simulink library "LimiterBtc"  (R2022b)
settings: Solver=VariableStepAuto  StartTime=0.0  StopTime=10.0  RelTol=1e-3
undefined symbols (not defined in the file or in its folder): Column
libraries: TuneVar x15, TOP x8, AudioStats x1, FeaturePath x1, HandyTextFile x1
settings Model: Creator=db1045444  LastModifiedBy=kl13806
settings SolverCC: AlgebraicLoopSolver=TrustRegion
settings DebuggingCC: UnconnectedInputMsg=warning  UnconnectedOutputMsg=warning  UnconnectedLineMsg=warning  SFMachineParentedDataDiag=warning
settings ModelReferenceCC: EnableRefExpFcnMdlSchedulingChecks=on
settings RTWCC: DLArmComputeVersion=19.05

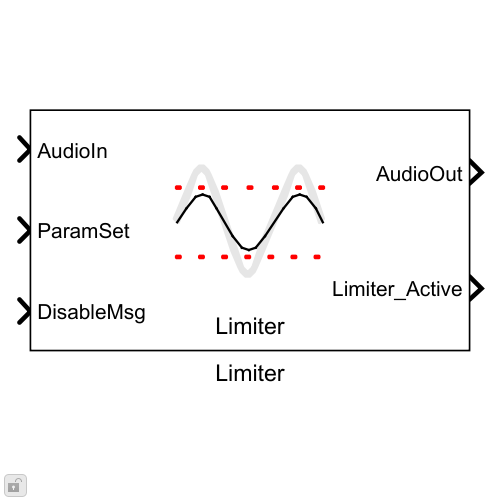
[thumbnail: Simulink's stored preview of the top-level diagram]
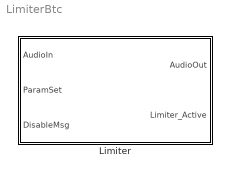
== system LimiterBtc ==
  Limiter : Subsystem  mask(Blocklib Limiter){Config=[], FeatureName=Limiter}
      mask prompts: Config "LimiterConfig"; FeatureName "Feature path name:"
      mask init:
      | blkh=gcbh;
      | Config=BTConfig.Assert(blkh,Config);
      | 
      | Config.Validate();
      | BTConfig.InitSetFeatureIfPresent(blkh,'FeatureName');
      mask Callback Config: BTConfig.CallbackHideIfPresent(gcbh,{'FeatureName'});
      mask TypeOptions FeatureName: FeaturePath/FeatureName
      mask Display:
      | [path,w,h] = IconLimiterMask();
      | 
      | % work in pixels since the icon does not scale
      | pos = get(gcbh,'position');
      | bw = pos(3) - pos(1);
      | bh = pos(4) - pos(2);
      | 
      | % Draw centered icon
      | xAdj = bw/2 - w/2;
      | yAdj = bh/2 - h/2 + 4;
      | for i=1:length(path)
      |     if (path(i).rgb(1) >= 0)
      |         patch(path(i).x+xAdj, path(i).y+yAdj, path(i).rgb);
      |     end
      |     if (path(i).stroke(1) >= 0)
      |         plot(path(i).x+xAdj, path(i).y+yAdj);
      |     end
      | end
      | 
      | % Display some text
      | text(bw/2, 4,FeatureName, ...
      |     'horizontalAlignment','center', ...
      |     'VerticalAlignment','bottom');

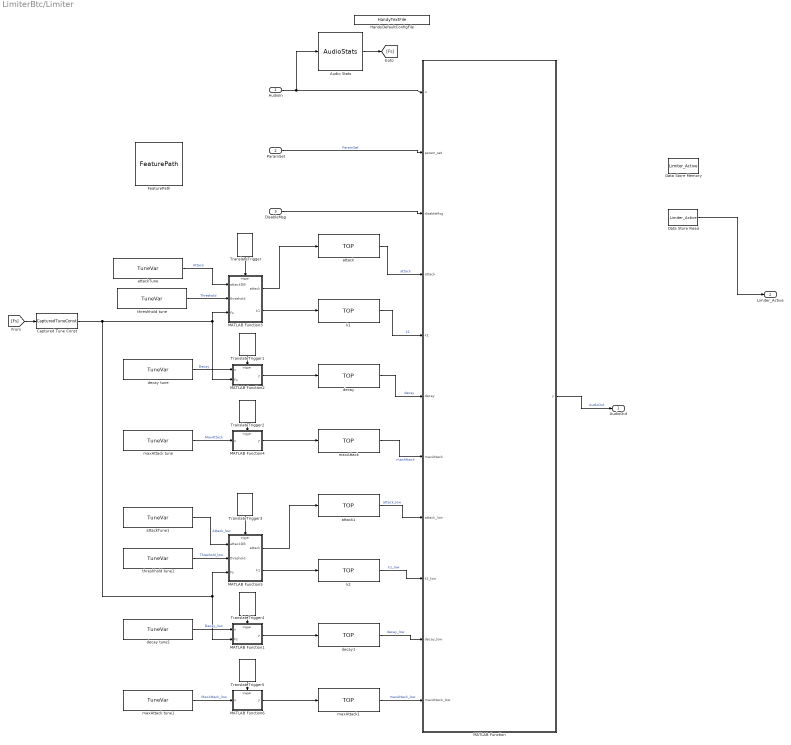
== system LimiterBtc/Limiter ==
  AudioIn : Inport
  ParamSet : Inport  Port=2
  DisableMsg : Inport  Port=3
  Audio Stats : AudioStats/AudioStats  DoSampleRate=on  TypeSampleRate=double  DoCallRate=off  TypeCallRate=Inherit: auto  DoFrameSize=off  TypeFrameSize=Inherit: auto  DoChannelCount=off  TypeChannelCount=single  DoTaskRateFactor=off  TypeTaskRateFactor=Inherit: auto  MacroNameRoot=AUDIO  MacroNameRootEval='AUDIO'  IsMacroNameEval=off  MacroSampleRate=off  MacroCallRate=off  MacroFrameSize=off  MacroChannelCount=off  MacroTaskRateFactor=off  MacroTaskId=off  ValidateSampleRate=off  ValueSampleRate=[]  ValidateCallRate=off  ValueCallRate=[]  ValidateFrameSize=off  ValueFrameSize=[]  ValidateChannelCount=off  ValueChannelCount=[]  ValidateTaskRateFactor=off  ValueTaskRateFactor=[]
      settings: SourceProductName=Bose Talaria
  Captured Tune Const : TuneVar/CapturedTuneConst  TriggerInit=[-235 487 -135 523]  Role=Automatic
      settings: SourceProductName=Bose Talaria
  Data Store Memory : DataStoreMemory  DataStoreName=Limiter_Active  ShowAdditionalParam=off  OutDataTypeStr=uint32
  Data Store Read : DataStoreRead  DataStoreName=Limiter_Active  IndexOptions=Index vector (dialog)  Indices=1  OutputSizes=1
  FeaturePath : FeaturePath/FeaturePath  FeatureName=Limiter  IsGroup=off  GroupNumber=-1  IsModule=off  TriggerInit=[10 64 125 171]
      settings: SourceProductName=Bose Talaria
  HandyDefaultConfigFile : HandyTextFile/HandyTextFile  TemplateSource=Config  FileSuffix=Init  OpenDialogOnLoad=off  UseThisBlockName=off  AddGrandParentNamePrefix=off  TheDefaultText=|  ShowInLibBrowser=on
      | % $(FILENAME) Setup model parameters for each "Init" callback (e.g. update diagram)
      | sample_rate_in_hertz = 44100;
      | frame_size = 32;
      | sysin_channel_count = 2;
      settings: SourceProductName=Bose Talaria
  MATLAB Function : MATLAB Function  TreatAsAtomicUnit=on
  MATLAB Function1 : MATLAB Function  TreatAsAtomicUnit=on
  MATLAB Function2 : MATLAB Function  TreatAsAtomicUnit=on
  MATLAB Function3 : MATLAB Function  TreatAsAtomicUnit=on
  MATLAB Function4 : MATLAB Function  TreatAsAtomicUnit=on
  MATLAB Function5 : MATLAB Function  TreatAsAtomicUnit=on
  MATLAB Function6 : MATLAB Function  TreatAsAtomicUnit=on
  TranslateTrigger : TuneVar/TranslateTrigger  TriggerInit=[261 290 299 345]
      settings: SourceProductName=Bose Talaria
  TranslateTrigger1 : TuneVar/TranslateTrigger  TriggerInit=[266 535 304 590]
      settings: SourceProductName=Bose Talaria
  TranslateTrigger2 : TuneVar/TranslateTrigger  TriggerInit=[266 700 304 755]
      settings: SourceProductName=Bose Talaria
  TranslateTrigger3 : TuneVar/TranslateTrigger  TriggerInit=[261 930 299 985]
      settings: SourceProductName=Bose Talaria
  TranslateTrigger4 : TuneVar/TranslateTrigger  TriggerInit=[266 1175 304 1230]
      settings: SourceProductName=Bose Talaria
  TranslateTrigger5 : TuneVar/TranslateTrigger  TriggerInit=[266 1340 304 1395]
      settings: SourceProductName=Bose Talaria
  attack : TOP/TOP  TriggerInit=[460 292 610 348]  TopName=attack  DataType=single  BankNumber=0  PreOverlay=false  PostOverlay=false  Role=Automatic
      settings: SourceProductName=Bose Talaria
  attack1 : TOP/TOP  TriggerInit=[460 932 610 988]  TopName=attack_low  DataType=single  BankNumber=0  PreOverlay=false  PostOverlay=false  Role=Automatic
      settings: SourceProductName=Bose Talaria
  attackTune : TuneVar/TuneVar  TuneName=Attack  SpecifyMaxSize=off  VariableDim=2 (Column)  MaxSize=[1 16]  TunabilityNumber=1  MinValue=[]  MaxValue=[]  TriggerInit=[-45 350 125 400]  MaskValue=Config.DefaultAttackDb
      settings: SourceProductName=Bose Talaria
  attackTune1 : TuneVar/TuneVar  TuneName=Attack_low  SpecifyMaxSize=off  VariableDim=2 (Column)  MaxSize=[1 1]  TunabilityNumber=1  MinValue=[]  MaxValue=[]  TriggerInit=[-20 965 150 1015]  MaskValue=Config.DefaultAttackLowDb
      settings: SourceProductName=Bose Talaria
  decay : TOP/TOP  TriggerInit=[460 612 610 668]  TopName=decay  DataType=single  BankNumber=0  PreOverlay=false  PostOverlay=false  Role=Automatic
      settings: SourceProductName=Bose Talaria
  decay tune : TuneVar/TuneVar  TuneName=Decay  SpecifyMaxSize=off  VariableDim=2 (Column)  MaxSize=[1 1]  TunabilityNumber=1  MinValue=[]  MaxValue=[]  TriggerInit=[-20 600 150 650]  MaskValue=Config.DefaultDecayDB
      settings: SourceProductName=Bose Talaria
  decay tune1 : TuneVar/TuneVar  TuneName=Decay_low  SpecifyMaxSize=off  VariableDim=2 (Column)  MaxSize=[1 1]  TunabilityNumber=1  MinValue=[]  MaxValue=[]  TriggerInit=[-20 1240 150 1290]  MaskValue=Config.DefaultDecayLowDb
      settings: SourceProductName=Bose Talaria
  decay1 : TOP/TOP  TriggerInit=[460 1252 610 1308]  TopName=decay_low  DataType=single  BankNumber=0  PreOverlay=false  PostOverlay=false  Role=Automatic
      settings: SourceProductName=Bose Talaria
  k1 : TOP/TOP  TriggerInit=[460 452 610 508]  TopName=k1  DataType=single  BankNumber=0  PreOverlay=false  PostOverlay=false  Role=Automatic
      settings: SourceProductName=Bose Talaria
  k2 : TOP/TOP  TriggerInit=[460 1092 610 1148]  TopName=k1_low  DataType=single  BankNumber=0  PreOverlay=false  PostOverlay=false  Role=Automatic
      settings: SourceProductName=Bose Talaria
  maxAttack : TOP/TOP  TriggerInit=[460 772 610 828]  TopName=maxAttack  DataType=single  BankNumber=0  PreOverlay=false  PostOverlay=false  Role=Automatic
      settings: SourceProductName=Bose Talaria
  maxAttack tune : TuneVar/TuneVar  TuneName=MaxAttack  SpecifyMaxSize=off  VariableDim=2 (Column)  MaxSize=[1 1]  TunabilityNumber=1  MinValue=[]  MaxValue=[]  TriggerInit=[-20 775 150 825]  MaskValue=Config.DefaultMaxAttackDb
      settings: SourceProductName=Bose Talaria
  maxAttack tune1 : TuneVar/TuneVar  TuneName=MaxAttack_low  SpecifyMaxSize=off  VariableDim=2 (Column)  MaxSize=[1 1]  TunabilityNumber=1  MinValue=[]  MaxValue=[]  TriggerInit=[-20 1415 150 1465]  MaskValue=Config.DefaultMaxAttackLowDb
      settings: SourceProductName=Bose Talaria
  maxAttack1 : TOP/TOP  TriggerInit=[460 1412 610 1468]  TopName=maxAttack_low  DataType=single  BankNumber=0  PreOverlay=false  PostOverlay=false  Role=Automatic
      settings: SourceProductName=Bose Talaria
  threshhold tune : TuneVar/TuneVar  TuneName=Threshold  SpecifyMaxSize=off  VariableDim=2 (Column)  MaxSize=[1 16]  TunabilityNumber=1  MinValue=[]  MaxValue=[]  TriggerInit=[-35 425 135 475]  MaskValue=Config.DefaultThreshold
      settings: SourceProductName=Bose Talaria
  threshhold tune1 : TuneVar/TuneVar  TuneName=Threshold_low  SpecifyMaxSize=off  VariableDim=2 (Column)  MaxSize=[1 1]  TunabilityNumber=1  MinValue=[]  MaxValue=[]  TriggerInit=[-20 1065 150 1115]  MaskValue=Config.DefaultThresholdLow
      settings: SourceProductName=Bose Talaria
  AudioOut : Outport  VectorParamsAs1DForOutWhenUnconnected=off
  Limiter_Active : Outport  Port=2
  wires:
  Data Store Read/1 -> Limiter_Active/1
  DisableMsg/1 -> MATLAB Function/3(disableMsg)
  AudioIn/1 -> Audio Stats/1, MATLAB Function/1(u)
  MATLAB Function/1(y) -> AudioOut/1  "AudioOut"
  attackTune/1 -> MATLAB Function3/1(attackDB)  "Attack"
  decay tune/1 -> MATLAB Function2/1(u)  "Decay"
  TranslateTrigger1/1 -> MATLAB Function2/Trigger
  attack/1 -> MATLAB Function/4(attack)  "attack"
  MATLAB Function2/1(y) -> decay/1
  decay/1 -> MATLAB Function/6(decay)  "decay"
  Audio Stats/1 -> [Fs]
  [Fs] -> Captured Tune Const/1
  threshhold tune/1 -> MATLAB Function3/2(threshold)  "Threshold"
  TranslateTrigger/1 -> MATLAB Function3/Trigger
  MATLAB Function3/2(k1) -> k1/1
  k1/1 -> MATLAB Function/5(k1)  "k1"
  maxAttack tune/1 -> MATLAB Function4/1(u)  "MaxAttack"
  TranslateTrigger2/1 -> MATLAB Function4/Trigger
  MATLAB Function4/1(y) -> maxAttack/1
  maxAttack/1 -> MATLAB Function/7(maxAttack)  "maxAttack"
  MATLAB Function3/1(attack) -> attack/1
  MATLAB Function5/1(attack) -> attack1/1
  maxAttack1/1 -> MATLAB Function/11(maxAttack_low)  "maxAttack_low"
  MATLAB Function6/1(y) -> maxAttack1/1
  TranslateTrigger5/1 -> MATLAB Function6/Trigger
  Captured Tune Const/1 -> MATLAB Function3/3(Fs), MATLAB Function2/2(Fs), MATLAB Function5/3(Fs), MATLAB Function1/2(Fs)
  MATLAB Function1/1(y) -> decay1/1
  decay1/1 -> MATLAB Function/10(decay_low)  "decay_low"
  decay tune1/1 -> MATLAB Function1/1(u)  "Decay_low"
  k2/1 -> MATLAB Function/9(k1_low)  "k1_low"
  attackTune1/1 -> MATLAB Function5/1(attackDB)  "Attack_low"
  threshhold tune1/1 -> MATLAB Function5/2(threshold)  "Threshold_low"
  MATLAB Function5/2(k1) -> k2/1
  TranslateTrigger3/1 -> MATLAB Function5/Trigger
  maxAttack tune1/1 -> MATLAB Function6/1(u)  "MaxAttack_low"
  TranslateTrigger4/1 -> MATLAB Function1/Trigger
  attack1/1 -> MATLAB Function/8(attack_low)  "attack_low"
  ParamSet/1 -> MATLAB Function/2(param_set)  "ParamSet"

== matlab function LimiterBtc/Limiter/MATLAB Function1 ==
  data: u input; y output; Fs input
  events: trigger input FUNCTION_CALL_EVENT
function y = fcn(u, Fs)

% Convert from dB to linear
y = single(undb20(abs(u.Value) / Fs));

== matlab function LimiterBtc/Limiter/MATLAB Function ==
  data: u input; param_set input; disableMsg input; y output; attack input; k1 input; decay input; maxAttack input; attack_low input; k1_low input; decay_low input; maxAttack_low input; Limiter_Active data_store_memory
function y = limiter(u, param_set, disableMsg, attack, k1, decay, maxAttack, attack_low, k1_low, decay_low, maxAttack_low)

% This is the main function for the Limiter.
% It takes an audio input, as well as 8 tunable variables (2 sets of 4),
% which are attack, maxAttack, k1, and decay. It will limit, or apply
% a gain reduction, to any samples that are essentially above a 
% pre-set threshold. 

% Grab data from input
y = coder.nullcopy(u);
[frame_size, channel_count] = size(u);

% Initialize memory
% attack = single(2.5768580901e-002 * ones(1,channel_count));
% decay = single(1.0002610981e+000 * ones(1,channel_count));
maxGain = single(1);
% maxAttack = single(3.1622776602e-001 * ones(1,channel_count));
% k1 = single(2.8631756556e-002 * ones(1,channel_count));

persistent state;
if isempty(state)
    state = single(1 * ones(1,channel_count));
end

if (param_set == 1)
    attack_param = attack;
    k1_param = k1;
    decay_param = decay;
    maxAttack_param = maxAttack;
else
    attack_param = attack_low;
    k1_param = k1_low;
    decay_param = decay_low;
    maxAttack_param = maxAttack_low;
end

global Limiter_Active;
Limiter_Active = uint32(0);
% Check for a disable RTC message, pass audio through unaffected if so
if (disableMsg)
    y(:) = u(:);
else
    % Process the audio
    for i = 1:channel_count
        k0 = 1 + attack_param(i);
        g1 = state(i);
        temp = single(0);
        temp1 = temp;
        for s = 1:frame_size
            % Compute the gain for this sample. Implementation copied from BDSP
            p1 = k1_param(i) * g1;
            p2 = u(s, i);
            p2 = abs(p2);
            temp = temp + p2;
            g1 = g1 * decay_param(i);
            p2 = p2 * p1;
            p2 = max(p2, attack_param(i));
            p2 = k0 - p2;
            p2 = max(p2, maxAttack_param(i));
            g1 = g1 * p2;
            g1 = min(g1, maxGain);
            % Apply the gain
            y(s, i) = u(s, i) * g1;
            p3 = abs(y(s,i));
            temp1 = temp1 + p3;
        end
        
        state(i) = g1;
        if temp1 < temp
            Limiter_Active  =  Limiter_Active + 2^(i-1);
        end
    end
end

== matlab function LimiterBtc/Limiter/MATLAB Function2 ==
  data: u input; y output; Fs input
  events: trigger input FUNCTION_CALL_EVENT
function y = fcn(u, Fs)

% Convert decay value from dB to linear
y = single(undb20(abs(u.Value) / Fs));

== matlab function LimiterBtc/Limiter/MATLAB Function3 ==
  data: attackDB input; threshold input; Fs input; attack output; k1 output
  events: trigger input FUNCTION_CALL_EVENT
function [attack, k1]= fcn(attackDB, threshold, Fs)

% This function translates threshold and attackDB into a k1 value
% k1 is used later in the main Limiter function to apply gain redux

% If we find that any channel has a threshold value of zero,
% reset it to 100, for we essentially do not want to limit 
% that specific channel.
minThreshold = 0.001;   % check against small number, set to zero if so. 
threshold.Value(threshold.Value < minThreshold) = 0;
if ~(all(threshold.Value))
    threshold.Value(find(threshold.Value == 0)) = 100;
end

% If we find attack value is 0, set to 10000
if ~(all(attackDB.Value))
    attackDB.Value(find(attackDB.Value == 0)) = 10000;
end

% Set output values
attack = single(1 - undb20(-abs(attackDB.Value) / Fs));
k1 = attack ./ single(threshold.Value);

== matlab function LimiterBtc/Limiter/MATLAB Function4 ==
  data: u input; y output
  events: trigger input FUNCTION_CALL_EVENT
function y = fcn(u)

% Translate from dB to linear
y = single(undb20(-abs(u.Value)));

== matlab function LimiterBtc/Limiter/MATLAB Function5 ==
  data: attackDB input; threshold input; Fs input; attack output; k1 output
  events: trigger input FUNCTION_CALL_EVENT
function [attack, k1]= fcn(attackDB, threshold, Fs)

% This function translates threshold and attackDB into a k1 value
% k1 is used later in the main Limiter function to apply gain redux

% If we find that any channel has a threshold value of zero,
% reset it to 100, for we essentially do not want to limit 
% that specific channel.
minThreshold = 0.001;   % check against small number, set to zero if so. 
threshold.Value(threshold.Value < minThreshold) = 0;
if ~(all(threshold.Value))
    threshold.Value(find(threshold.Value == 0)) = 100;
end

% If we find attack value is 0, set to 10000
if ~(all(attackDB.Value))
    attackDB.Value(find(attackDB.Value == 0)) = 10000;
end

% Set output values
attack = single(1 - undb20(-abs(attackDB.Value) / Fs));
k1 = attack ./ single(threshold.Value);

== matlab function LimiterBtc/Limiter/MATLAB Function6 ==
  data: u input; y output
  events: trigger input FUNCTION_CALL_EVENT
function y = fcn(u)

% Convert from dB to linear
y = single(undb20(-abs(u.Value)));
